simulink model "c_code_using_MATLAB_fn"  (R2018b)
settings: Solver=VariableStepAuto  StartTime=0.0  StopTime=10.0  RelTol=1e-3
libraries: simulink x2
settings Model: Creator=marwan  LastModifiedBy=marwan
settings SFSimCC: SimCustomHeaderCode="#include \"MATLAB_proj/add_lib.h\""  SimUserSources=MATLAB_proj/main.c

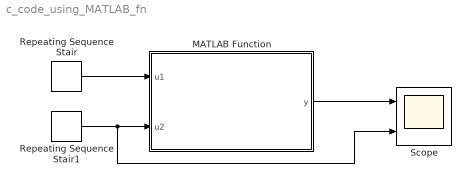
== system c_code_using_MATLAB_fn ==
  MATLAB Function : MATLAB Function  TreatAsAtomicUnit=on
  Repeating Sequence Stair : simulink/Sources/Repeating Sequence Stair  OutValues=[1 2 3 4 5 6].'  tsamp=-1  OutMin=[]  OutMax=[]  OutDataTypeStr=double  OutputDataTypeScalingMode=double  OutDataType=fixdt(0,8)  ConRadixGroup=Best Precision: Vector-wise  OutScaling=2^-12
  Repeating Sequence Stair1 : simulink/Sources/Repeating Sequence Stair  OutValues=[1 2 3 4 5 6].'  tsamp=-1  OutMin=[]  OutMax=[]  OutDataTypeStr=double  OutputDataTypeScalingMode=double  OutDataType=fixdt(0,8)  ConRadixGroup=Best Precision: Vector-wise  OutScaling=2^-12
  Scope : Scope  NumInputPorts=2
  wires:
  Repeating Sequence Stair/1 -> MATLAB Function/1(u1)
  Repeating Sequence Stair1/1 -> Scope/2, MATLAB Function/2(u2)
  MATLAB Function/1(y) -> Scope/1

== matlab function c_code_using_MATLAB_fn/MATLAB Function ==
  data: u1 input; y output; u2 input
function y = fcn(u1,u2)
    y=0.0;
y = coder.ceval('add_2',u1,u2);
